simulink model "Exemplo_Submarino"  (R2015a)
settings: Solver=ode3  StartTime=0.0  StopTime=1000  FixedStep=0.1  MaxStep=1e-4  RelTol=1e-3
libraries: AvgModels x3, simulink x2
settings Model: CovSFcnEnable=off  Creator=luigi  LastModifiedBy=lgalo
settings DebuggingCC: FcnCallInpInsideContextMsg=EnableAllAsWarning
settings GRTTargetCC: CombineOutputUpdateFcns=off  GRTInterface=on

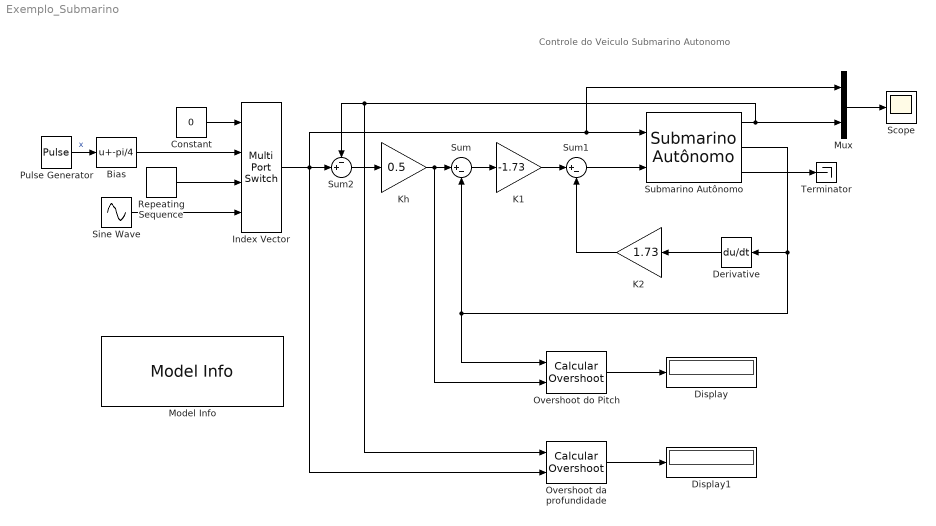
== system Exemplo_Submarino ==
  note: Controle do Veiculo Submarino Autonomo
  Bias : Bias  Bias=-pi/4
  Constant : Constant  Value=0
  Derivative : Derivative
  Display : Display
  Display1 : Display
  Index Vector : MultiPortSwitch  DataPortOrder=Zero-based contiguous  zeroidx=on
  K1 : Gain  Gain=-1.73
  K2 : Gain  Gain=1.73
  Kh : Gain  Gain=0.5
  Model Info : simulink/Model-Wide Utilities/Model Info  BlockCM=none  Frame=on  DisplayStringWithTags=|  HorizontalTextAlignment=Center  LeftAlignmentValue=0.5  SourceBlockDiagram=Exemplo_Submarino  TagMaxNumber=20
      | Model Info
      | %<ModelName>
      | Criado: %<Created>
      | %<Creator>
      | Atualizado: %<LastModificationDate>
  Mux : Mux  Inputs=2
  Overshoot da profundidade : AvgModels/Calcular Overshoot
  Overshoot do Pitch : AvgModels/Calcular Overshoot
  Pulse Generator : DiscretePulseGenerator  PulseType=Time based  Amplitude=pi/2  Period=300  PulseWidth=50
  Repeating Sequence : simulink/Sources/Repeating Sequence  rep_seq_t=[0 100 200]  rep_seq_y=[-1 1 -1]*4
  Scope : Scope
  Sine Wave : Sin  Frequency=0.2  SampleTime=0
  Submarino Autônomo : AvgModels/Modelos Animados/Submarino Autônomo
  Sum : Sum  Inputs=|+-
  Sum1 : Sum  Inputs=|+-
  Sum2 : Sum  Inputs=-+|
  Terminator : Terminator
  wires:
  K1/1 -> Sum1/1
  Sum1/1 -> Submarino Autônomo/2
  Index Vector/1 -> Overshoot da profundidade/2, Sum2/2, Mux/1, Submarino Autônomo/1
  Sum/1 -> K1/1
  Submarino Autônomo/2 -> Overshoot do Pitch/1, Sum/2, Derivative/1
  Mux/1 -> Scope/1
  K2/1 -> Sum1/2
  Derivative/1 -> K2/1
  Pulse Generator/1 -> Bias/1  "x"
  Constant/1 -> Index Vector/1
  Sine Wave/1 -> Index Vector/4
  Repeating Sequence/1 -> Index Vector/3
  Bias/1 -> Index Vector/2
  Submarino Autônomo/1 -> Mux/2, Overshoot da profundidade/1, Sum2/1
  Sum2/1 -> Kh/1
  Kh/1 -> Overshoot do Pitch/2, Sum/1
  Overshoot do Pitch/1 -> Display/1
  Overshoot da profundidade/1 -> Display1/1
  Submarino Autônomo/3 -> Terminator/1
